simulink model "divisore"  (R2023b)
settings: Solver=FixedStepAuto  StartTime=0.0  StopTime=10  FixedStep=0.001  RelTol=1e-3
libraries: simulink x1
settings Model: Creator=stefa  LastModifiedBy=stefa

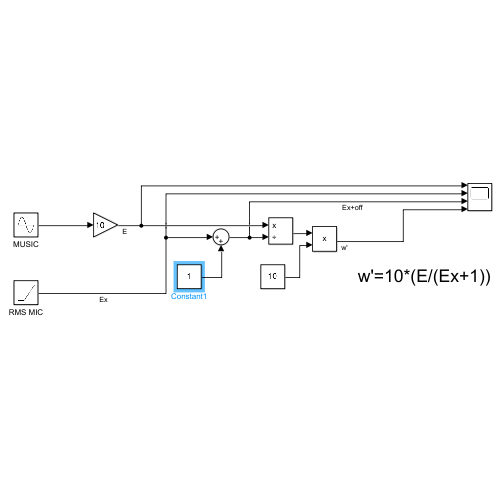
[thumbnail: Simulink's stored preview of the top-level diagram]
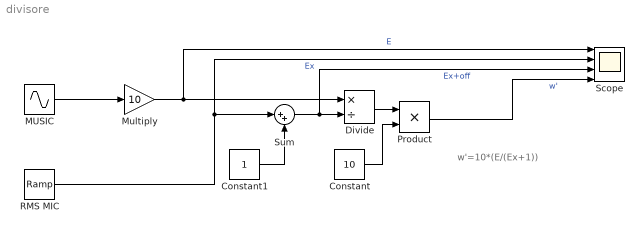
== system divisore ==
  note: w'=10*(E/(Ex+1))
  Constant : Constant  Value=10
  Constant1 : Constant
  Divide : Product  Inputs=*/  RndMeth=Zero  SaturateOnIntegerOverflow=on
  MUSIC : Sin  Amplitude=0.1  Frequency=10  SampleTime=0
  Multiply : Gain  Gain=10
  Product : Product
  RMS MIC : simulink/Sources/Ramp  slope=0.7  start=0  InitialOutput=0
  Scope : Scope  NumInputPorts=4
  Sum : Sum  Inputs=|++
  wires:
  MUSIC/1 -> Multiply/1
  Multiply/1 -> Scope/1, Divide/1  "E"
  RMS MIC/1 -> Sum/1, Scope/2  "Ex"
  Constant/1 -> Product/2
  Constant1/1 -> Sum/2
  Divide/1 -> Product/1
  Sum/1 -> Scope/3, Divide/2  "Ex+off"
  Product/1 -> Scope/4  "w'"
